simulink model "CLF_CBF_Unified"  (R2024b)
settings: Solver=ode45  StartTime=0.0  StopTime=60  RelTol=1e-6  AbsTol=1e-8
libraries: simulink_extras x6
settings Model: Creator=LAPTOPASADI  LastModifiedBy=LAPTOPASADI

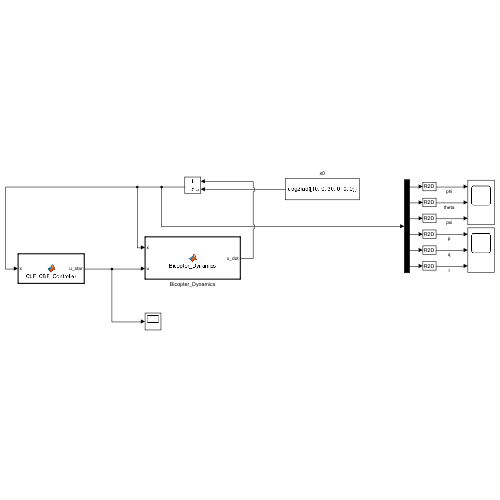
[thumbnail: Simulink's stored preview of the top-level diagram]
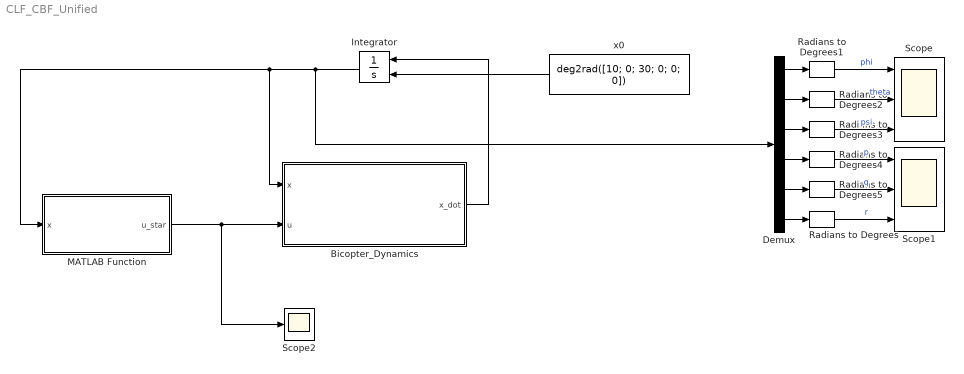
== system CLF_CBF_Unified ==
  Bicopter_Dynamics : MATLAB Function  TreatAsAtomicUnit=on
  Demux : Demux  Outputs=6
  Integrator : Integrator  InitialConditionSource=external
  MATLAB Function : MATLAB Function  TreatAsAtomicUnit=on
  Radians to Degrees{,1..5} (6 alike) : simulink_extras/Transformations/Radians to Degrees
  Scope : Scope  NumInputPorts=3
  Scope1 : Scope  NumInputPorts=3
  Scope2 : Scope
  x0 : Constant  Value=deg2rad([10; 0; 30; 0; 0; 0])  VectorParams1D=off  OutDataTypeStr=double
  wires:
  Demux/1 -> Radians to Degrees1/1
  Demux/2 -> Radians to Degrees2/1
  Demux/5 -> Radians to Degrees5/1
  Demux/6 -> Radians to Degrees/1
  Demux/3 -> Radians to Degrees3/1
  Demux/4 -> Radians to Degrees4/1
  Radians to Degrees1/1 -> Scope/1  "phi"
  Radians to Degrees2/1 -> Scope/2  "theta"
  Radians to Degrees3/1 -> Scope/3  "psi"
  Radians to Degrees4/1 -> Scope1/1  "p"
  Radians to Degrees5/1 -> Scope1/2  "q"
  Radians to Degrees/1 -> Scope1/3  "r"
  Integrator/1 -> Demux/1, MATLAB Function/1(x), Bicopter_Dynamics/1(x)
  MATLAB Function/1(u_star) -> Scope2/1, Bicopter_Dynamics/2(u)
  x0/1 -> Integrator/2
  Bicopter_Dynamics/1(x_dot) -> Integrator/1

== matlab function CLF_CBF_Unified/Bicopter_Dynamics ==
  data: x input; u input; x_dot output
function x_dot = Bicopter_Dynamics(x, u)
%% --- System Parameters ---
Ixx = 0.0043;  Iyy = 0.0142;  Izz = 0.0176;  Ixz = 0.0001;
I   = [Ixx, 0, -Ixz;
       0,   Iyy, 0;
      -Ixz, 0,   Izz];

dcg      = 0.175;
hcg      = 0.085;
d_over_b = 1.2e-6 / 3.13e-5;

B_alloc = [0,  0,    dcg,      d_over_b;
           0,  hcg,  0,        0;
           0,  0,    d_over_b, -dcg];

%% --- Extract States ---
phi   = x(1);
theta = x(2);
p     = x(4);
q     = x(5);
r     = x(6);

omega = [p; q; r];

%% --- Euler Rate Matrix J(phi, theta) ---
cth = cos(theta);
if abs(cth) < 1e-6
    cth = sign(cth + 1e-6) * 1e-6;
end
J = [1,  sin(phi)*sin(theta)/cth,  cos(phi)*sin(theta)/cth;
     0,  cos(phi),                 -sin(phi);
     0,  sin(phi)/cth,              cos(phi)/cth];

%% --- State Derivative ---
euler_dot = J * omega;                          % phi_dot, theta_dot, psi_dot
tau_gyro  = -cross(omega, I * omega);           % gyroscopic torque
omega_dot = I \ (tau_gyro + B_alloc * u);       % angular acceleration

x_dot = [euler_dot; omega_dot];               
end

== matlab function CLF_CBF_Unified/MATLAB Function ==
  data: x input; u_star output
function u_star = CLF_CBF_Controller(x)
% CLF_CBF_CONTROLLER
%% --- Parameters ---
Ixx = 0.0043;  Iyy = 0.0142;  Izz = 0.0176;  Ixz = 0.0001;
I   = [Ixx, 0, -Ixz;
       0,   Iyy, 0;
      -Ixz, 0,   Izz];

dcg      = 0.175;
hcg      = 0.085;
d_over_b = 1.2e-6 / 3.13e-5;

B_alloc = [0,  0,    dcg,      d_over_b;
           0,  hcg,  0,        0;
           0,  0,    d_over_b, -dcg];

gamma     = 0.5;
p_penalty = 1e4;
u_min     = -0.1;
u_max     =  0.1;
theta_max = deg2rad(20);
alpha1    = 5;
alpha2    = 5;

%% --- P matrix ---

P = [0.11250,       0,       0,   0.01250,       0,       0;
          0,  0.11250,       0,         0,  0.01250,       0;
          0,       0,  0.11250,         0,       0,  0.01250;
     0.01250,      0,       0,   0.01563,       0,       0;
          0,  0.01250,      0,         0,  0.01563,       0;
          0,       0,  0.01250,         0,       0,  0.01563];

%% --- Extract States ---
phi   = x(1);  theta = x(2);  psi = x(3);
p     = x(4);  q     = x(5);  r   = x(6);
omega = [p; q; r];
y     = [phi; theta - deg2rad(30); psi];

%% --- CLF ---
J     = uni_J(phi, theta);
y_dot = J * omega;
eta   = [y; y_dot];
V     = eta' * P * eta;

if V < 1e-8
    u_star = zeros(4,1);
    return;
end

Jdot        = uni_Jdot(phi, theta, omega);
tau_gyro    = -cross(omega, I * omega);
omega_drift = I \ tau_gyro;

alpha_vec = Jdot * omega + J * omega_drift;
A_mat     = J * (I \ B_alloc);

f_eta   = [y_dot;      alpha_vec];
g_eta   = [zeros(3,4); A_mat   ];
dV_deta = 2 * eta' * P;
LfV     = dV_deta * f_eta;
LgV     = dV_deta * g_eta;

%% --- CBF: HOCBF pitch (h = theta_max - theta) ---
J2        = [0,  cos(phi),  -sin(phi)];
theta_dot = J2 * omega;
psi0      = theta_max - theta;
psi1      = -theta_dot + alpha1 * psi0;

gyro     = I \ cross(omega, I * omega);
Lf_psi1  = J2 * gyro + alpha1 * theta_dot;
Lg_psi1  = -J2 * (I \ B_alloc);

%% --- Unified QP: z = [u(4x1); delta] ---
H   = 2 * diag([1, 1, 1, 1, p_penalty]);
fqp = zeros(5,1);

A_clf = [LgV,      -1];   
b_clf = -LfV - gamma * V;

A_cbf = [-Lg_psi1,  0];   
b_cbf =  Lf_psi1 + alpha2 * psi1;

Aineq = [A_clf; A_cbf];
bineq = [b_clf; b_cbf];
lb    = [u_min*ones(4,1); 0  ];
ub    = [u_max*ones(4,1); Inf];

opts = optimoptions('quadprog', 'Algorithm', 'active-set', 'Display', 'off', 'MaxIterations', 200);
z    = quadprog(H, fqp, Aineq, bineq, [], [], lb, ub, zeros(5,1), opts);


if isempty(z)
    u_star = zeros(4,1);
else
    u_star = z(1:4);
end
end

%%  Local helpers
function J = uni_J(phi, theta)
    cth = cos(theta);
    if abs(cth) < 1e-6,  cth = sign(cth+1e-6)*1e-6;  end
    J = [1,  sin(phi)*sin(theta)/cth,  cos(phi)*sin(theta)/cth;
         0,  cos(phi),                 -sin(phi);
         0,  sin(phi)/cth,              cos(phi)/cth];
end

function Jd = uni_Jdot(phi, theta, omega)
    J  = uni_J(phi, theta);
    ed = J * omega;
    pd = ed(1);  td = ed(2);
    cth = cos(theta);  sth = sin(theta);
    if abs(cth) < 1e-6,  cth = sign(cth+1e-6)*1e-6;  end
    tth = sth/cth;  sc = 1/cth;  s2 = sc^2;
    dJdphi   = [0,  cos(phi)*tth,       -sin(phi)*tth;
                0, -sin(phi),            -cos(phi);
                0,  cos(phi)*sc,         -sin(phi)*sc];
    dJdtheta = [0,  sin(phi)*s2,          cos(phi)*s2;
                0,  0,                    0;
                0,  sin(phi)*sc*tth,      cos(phi)*sc*tth];
    Jd = dJdphi*pd + dJdtheta*td;
end
